simulink model "model"  (R2025b)
settings: Solver=FixedStepAuto  StartTime=0.0  StopTime=inf  FixedStep=0.01  RelTol=1e-3  EnableMultiTasking=on
libraries: GenericTarget x18, simulink x3
settings Model: Creator=Scythe  LastModifiedBy=damerius
settings SolverCC: ConcurrentTasks=on
settings DataIOCC: SaveOutput=off  SignalLogging=off  DSMLogging=off  SaveTime=off  ReturnWorkspaceOutputs=off
settings OptimizationCC: DefaultParameterBehavior=Inlined  EnhancedBackFolding=on  PassReuseOutputArgsAs=Individual arguments  ZeroExternalMemoryAtStartup=off  ZeroInternalMemoryAtStartup=off  SimCompilerOptimization=on  OptimizeBlockOrder=speed  DifferentSizesBufferReuse=on  OptimizationCustomize=off  EfficientTunableParamExpr=on
settings DebuggingCC: ParameterTunabilityLossMsg=error  UnconnectedInputMsg=warning  UnconnectedOutputMsg=warning  UnconnectedLineMsg=warning
settings HardwareCC: ProdBitPerLong=64.0  ProdHWDeviceType=Intel->x86-64 (Linux 64)  TargetBitPerLong=64.0  TargetBitPerPointer=64.0  TargetBitPerSizeT=64.0  TargetBitPerPtrDiffT=64.0  TargetLargestAtomicFloat=Float  TargetIntDivRoundTo=Zero  TargetEndianess=LittleEndian  TargetWordSize=64.0  TargetHWDeviceType=Intel->x86-64 (Linux 64)  ProdEqTarget=off
settings ModelReferenceCC: EnableRefExpFcnMdlSchedulingChecks=on
settings SFSimCC: SimGenImportedTypeDefs=on  SimTargetLang=C++  SimDLTargetLibrary=mkl-dnn
settings RTWCC: SystemTargetFile=ert.tlc  GenCodeOnly=on  PackageGeneratedCodeAndArtifacts=on  PackageName=PackNGo  TemplateMakefile=ert_default_tmf  Toolchain=CMake  DataTypeReplacement=CDataTypesFixedWidth  TargetLang=C++  Description=Embedded Coder
settings CodeAppCC: ForceParamTrailComments=on  IgnoreCustomStorageClasses=off  MaxIdLength=128.0  OperatorAnnotations=on  SimulinkDataObjDesc=on  SFDataObjDesc=on  InsertBlockDesc=on  StateflowObjectComments=on  MATLABSourceComments=on  UseSimReservedNames=on
settings ERTTargetCC: TargetOS=NativeThreadsExample  RootIOFormat=Structure reference  ERTCustomFileTemplate=example_file_process.tlc  IndentSize=4  NewlineStyle=LF  MaxLineWidth=256.0  MaxIdInt64=INT64_MAX  MinIdInt64=INT64_MIN  MaxIdUint64=UINT64_MAX  MaxIdInt32=INT32_MAX  MinIdInt32=INT32_MIN  MaxIdUint32=UINT32_MAX  MaxIdInt16=INT16_MAX  MinIdInt16=INT16_MIN  MaxIdUint16=UINT16_MAX  MaxIdInt8=INT8_MAX  MinIdInt8=INT8_MIN  MaxIdUint8=UINT8_MAX  DynamicArrayContainerType=coder::array  TargetLangStandard=C++20 (ISO)  CodeInterfacePackaging=C++ class  SubcomponentCodeInterfacePackaging=C++ class  SupportContinuousTime=on  SupportVariableSizeSignals=on

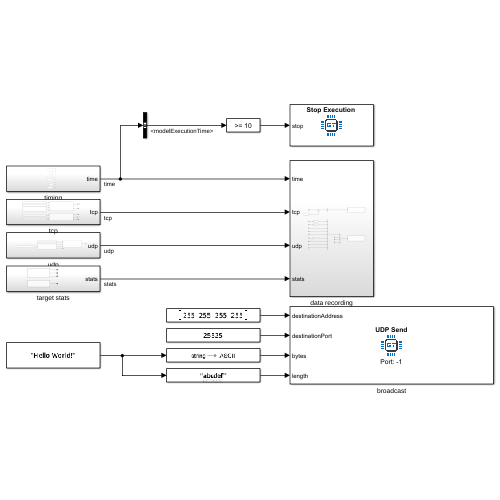
[thumbnail: Simulink's stored preview of the top-level diagram]
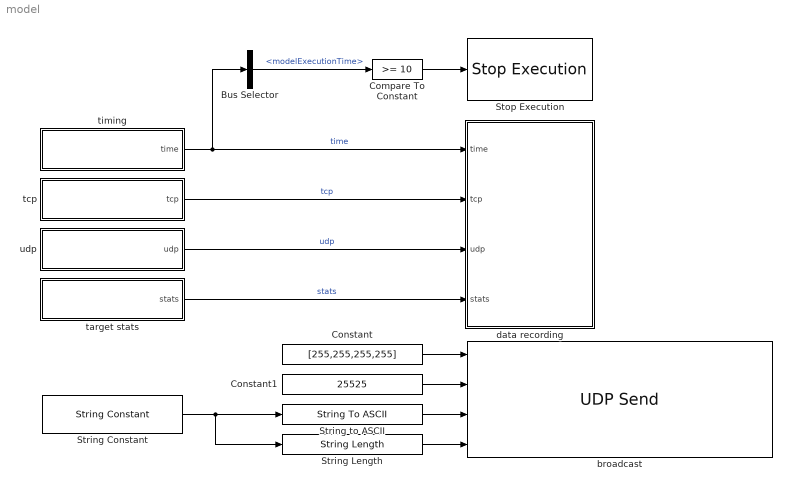
== system model ==
  Bus Selector : BusSelector  OutputSignals=modelExecutionTime
  Compare To Constant : simulink/Logic and Bit Operations/Compare To Constant  relop=>=  const=10  OutDataTypeStr=boolean
  Constant : Constant  Value=[255,255,255,255]  OutDataTypeStr=uint8
  Constant1 : Constant  Value=25525  OutDataTypeStr=uint16
  Stop Execution : GenericTarget/Interface/Stop Execution  SampleTime=0.01
      settings: SourceProductName=Generic Target
  String Constant : StringConstant  String="\"Hello World!\""
  String Length : StringLength  OutDataTypeStr=int32
  String to ASCII : StringToASCII  OutputVectorSize=63
  broadcast : GenericTarget/Interface/UDP Send  showDetails=off  localPort=-1  deviceName=''  multicastTTL=1  multicastInterfaceAddress=[0,0,0,0]  multicastAll=on  multicastLoop=on  socketPriority=6  allowBroadcast=on  allowZeroLengthMessage=off  SampleTime=1
      settings: SourceProductName=Generic Target
  data recording : Subsystem
  target stats : Subsystem
  tcp : Subsystem
  timing : Subsystem
  udp : Subsystem
  wires:
  target stats/1(stats) -> data recording/4(stats)  "stats"
  udp/1(udp) -> data recording/3(udp)  "udp"
  Bus Selector/1 -> Compare To Constant/1  "<modelExecutionTime>"
  timing/1(time) -> Bus Selector/1, data recording/1(time)  "time"
  Compare To Constant/1 -> Stop Execution/1
  Constant/1 -> broadcast/1
  Constant1/1 -> broadcast/2
  String to ASCII/1 -> broadcast/3
  String Length/1 -> broadcast/4
  String Constant/1 -> String Length/1, String to ASCII/1
  tcp/1(tcp) -> data recording/2(tcp)  "tcp"

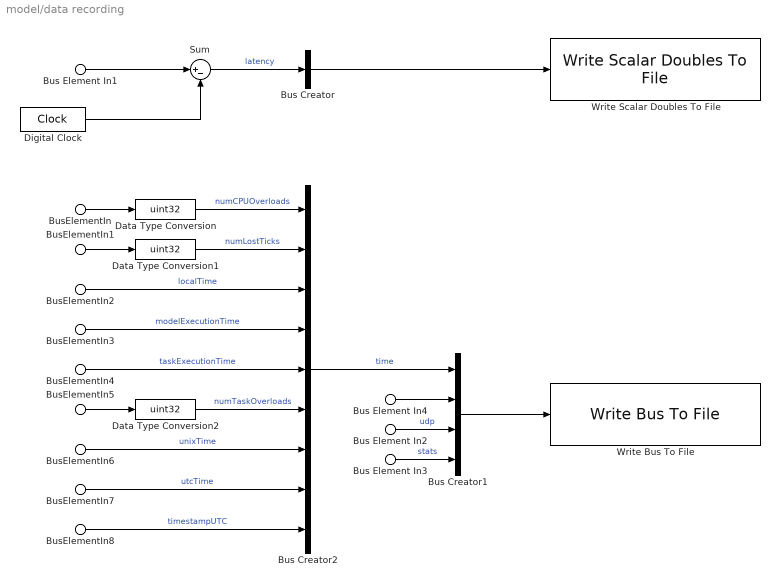
== system model/data recording ==
  Bus Element In1 : Inport  PortName=time  Element=modelExecutionTime
  BusElementIn3 : Inport  PortName=time  Element=modelExecutionTime
  BusElementIn : Inport  PortName=time  Element=numCPUOverloads
  BusElementIn1 : Inport  PortName=time  Element=numLostTicks
  BusElementIn2 : Inport  PortName=time  Element=localTime
  BusElementIn4 : Inport  PortName=time  Element=taskExecutionTime
  BusElementIn5 : Inport  PortName=time  Element=numTaskOverloads
  BusElementIn6 : Inport  PortName=time  Element=unixTime
  BusElementIn7 : Inport  PortName=time  Element=utcTime
  BusElementIn8 : Inport  PortName=time  Element=timestampUTC
  Bus Element In4 : Inport  Port=2  PortName=tcp
  Bus Element In2 : Inport  Port=3  PortName=udp
  Bus Element In3 : Inport  Port=4  PortName=stats
  Bus Creator : BusCreator  Inputs=1
  Bus Creator1 : BusCreator  Inputs=4
  Bus Creator2 : BusCreator  Inputs=9
  Data Type Conversion : DataTypeConversion  OutDataTypeStr=uint32  SaturateOnIntegerOverflow=off  RndMeth=Floor
  Data Type Conversion1 : DataTypeConversion  OutDataTypeStr=uint32  SaturateOnIntegerOverflow=off  RndMeth=Floor
  Data Type Conversion2 : DataTypeConversion  OutDataTypeStr=uint32  SaturateOnIntegerOverflow=off  RndMeth=Floor
  Digital Clock : DigitalClock  SampleTime=0.01
  Sum : Sum  Inputs=|+-
  Write Bus To File : GenericTarget/Interface/Write Bus To File  strID='bus'  numSamplesPerFile=0  threadPriority=30  writeFilesDuringSimulation=off  SampleTime=0.01  numBytesPerSample=305  strSignalNames='time.numCPUOverloads,time.numLostTicks,time.localTime.nanoseconds,time.localTime.second,time.localTime.minute,time.localTime.hour,time.localTime.mday,time.localTime.month,time.localTime.year,time.localTime.wday,time.localTime.yday,time.localTime.isdst,time.modelExecutionTime,time.taskExecutionTime,time.numTaskOverloads,time.unixTime,time.utcTime.nanoseconds,time.utcTime.second,time.utcTime.minute,time.utcTime.hour,time.utcTime.mday,time.utcTime.month,time.utcTime.year,time.utcTime.wday,time.utcTime.yday,time.utcTime.isdst,time.timestampUTC,tcp.tx_details.result,tcp.tx_details.lastErrorCode,tcp.tx_details.isConnected,tcp.rx_byte,tcp.rx_details.result,tcp.rx_details.lastErrorCode,tcp.rx_details.isConnected,udp.rx_details.sourceAddress,udp.rx_details.sourcePort,udp.rx_details.result,udp.rx_details.lastErrorCode,udp.tx_details.result,udp.tx_details.lastErrorCode,stats.applicationArguments.args,stats.applicationArguments.numCharacters,stats.applicationArguments.numArguments,stats.thermalZones'  strlenSignalNames=1002  strDimensions='[1],[1],[1],[1],[1],[1],[1],[1],[1],[1],[1],[1],[1],[1],[1],[1],[1],[1],[1],[1],[1],[1],[1],[1],[1],[1],[1],[1],[1],[1],[1],[1],[1],[1],[4],[1],[1],[1],[1],[1],[32 2],[2],[1],[8]'  strlenDimensions=178  strDataTypes='uint32,uint32,int32,int32,int32,int32,int32,int32,int32,int32,int32,int32,double,double,uint32,double,int32,int32,int32,int32,int32,int32,int32,int32,int32,int32,double,int32,int32,boolean,uint8,int32,int32,boolean,uint8,uint16,int32,int32,int32,int32,uint8,uint32,uint32,double'  strlenDataTypes=278
      settings: SourceProductName=Generic Target
  Write Scalar Doubles To File : GenericTarget/Interface/Write Scalar Doubles To File  strID='scalar_doubles'  numSamplesPerFile=0  threadPriority=30  writeFilesDuringSimulation=off  numSignals=1  signalNames=latency  numCharacters=7  SampleTime=0.01
      settings: SourceProductName=Generic Target
  wires:
  Bus Element In3/1 -> Bus Creator1/4  "stats"
  Bus Element In2/1 -> Bus Creator1/3  "udp"
  Bus Creator2/1 -> Bus Creator1/1  "time"
  BusElementIn8/1 -> Bus Creator2/9  "timestampUTC"
  BusElementIn7/1 -> Bus Creator2/8  "utcTime"
  BusElementIn6/1 -> Bus Creator2/7  "unixTime"
  Data Type Conversion2/1 -> Bus Creator2/6  "numTaskOverloads"
  BusElementIn4/1 -> Bus Creator2/5  "taskExecutionTime"
  BusElementIn3/1 -> Bus Creator2/4  "modelExecutionTime"
  BusElementIn2/1 -> Bus Creator2/3  "localTime"
  Data Type Conversion1/1 -> Bus Creator2/2  "numLostTicks"
  Data Type Conversion/1 -> Bus Creator2/1  "numCPUOverloads"
  BusElementIn5/1 -> Data Type Conversion2/1
  BusElementIn1/1 -> Data Type Conversion1/1
  BusElementIn/1 -> Data Type Conversion/1
  Bus Creator1/1 -> Write Bus To File/1
  Bus Creator/1 -> Write Scalar Doubles To File/1
  Sum/1 -> Bus Creator/1  "latency"
  Digital Clock/1 -> Sum/2
  Bus Element In1/1 -> Sum/1
  Bus Element In4/1 -> Bus Creator1/2

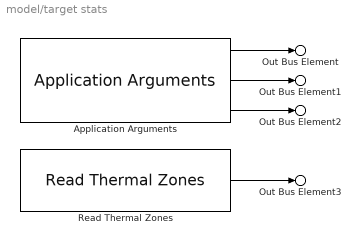
== system model/target stats ==
  Application Arguments : GenericTarget/Target Stats/Application Arguments  maxNumCharsPerArgument=32  maxNumArguments=2  SampleTime=0.01
      settings: SourceProductName=Generic Target
  Read Thermal Zones : GenericTarget/Target Stats/Read Thermal Zones  maxNumThermalZones=8  SampleTime=0.01
      settings: SourceProductName=Generic Target
  Out Bus Element : Outport  PortName=stats  Element=applicationArguments.args
  Out Bus Element1 : Outport  PortName=stats  Element=applicationArguments.numCharacters
  Out Bus Element2 : Outport  PortName=stats  Element=applicationArguments.numArguments
  Out Bus Element3 : Outport  PortName=stats  Element=thermalZones
  wires:
  Read Thermal Zones/1 -> Out Bus Element3/1
  Application Arguments/3 -> Out Bus Element2/1
  Application Arguments/2 -> Out Bus Element1/1
  Application Arguments/1 -> Out Bus Element/1

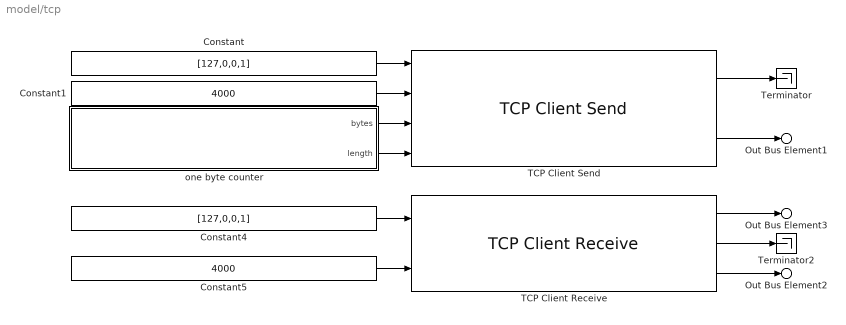
== system model/tcp ==
  Constant : Constant  Value=[127,0,0,1]  OutDataTypeStr=uint8
  Constant1 : Constant  Value=4000  OutDataTypeStr=uint16
  Constant4 : Constant  Value=[127,0,0,1]  OutDataTypeStr=uint8
  Constant5 : Constant  Value=4000  OutDataTypeStr=uint16
  TCP Client Receive : GenericTarget/Interface/TCP Client Receive  showDetails=on  manageConnection=off  localPort=0  deviceName=''  rxBufferSize=1  socketPriority=6  SampleTime=0.01
  TCP Client Send : GenericTarget/Interface/TCP Client Send  showDetails=on  manageConnection=on  localPort=0  deviceName=''  socketPriority=6  SampleTime=0.01
  Terminator : Terminator
  Terminator2 : Terminator
  one byte counter : Subsystem
  Out Bus Element1 : Outport  PortName=tcp  Element=tx_details
  Out Bus Element3 : Outport  PortName=tcp  Element=rx_byte
  Out Bus Element2 : Outport  PortName=tcp  Element=rx_details
  wires:
  TCP Client Send/2 -> Out Bus Element1/1
  Constant/1 -> TCP Client Send/1
  Constant1/1 -> TCP Client Send/2
  TCP Client Send/1 -> Terminator/1
  TCP Client Receive/1 -> Out Bus Element3/1
  TCP Client Receive/2 -> Terminator2/1
  Constant5/1 -> TCP Client Receive/2
  Constant4/1 -> TCP Client Receive/1
  TCP Client Receive/3 -> Out Bus Element2/1
  one byte counter/1(bytes) -> TCP Client Send/3
  one byte counter/2(length) -> TCP Client Send/4

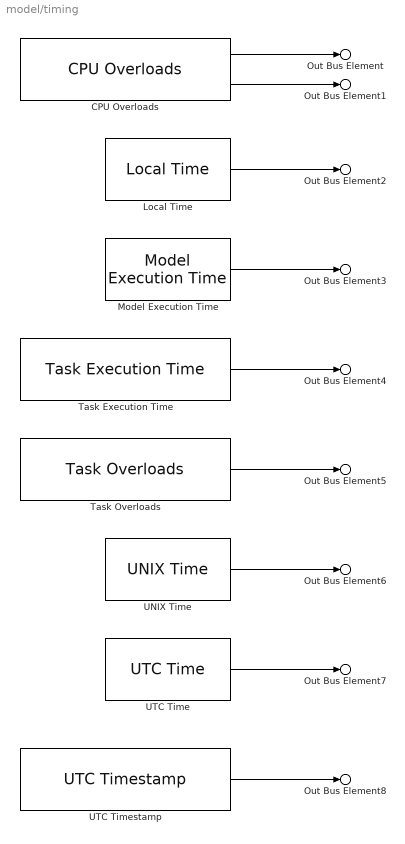
== system model/timing ==
  CPU Overloads : GenericTarget/Time/CPU Overloads  SampleTime=0.01
      settings: SourceProductName=Generic Target
  Local Time : GenericTarget/Time/Local Time  SampleTime=0.01
      settings: SourceProductName=Generic Target
  Model Execution Time : GenericTarget/Time/Model Execution Time  SampleTime=0.01
      settings: SourceProductName=Generic Target
  Task Execution Time : GenericTarget/Time/Task Execution Time  strTaskName='D1'  SampleTime=0.01
      settings: SourceProductName=Generic Target
  Task Overloads : GenericTarget/Time/Task Overloads  strTaskName='D1'  SampleTime=0.01
      settings: SourceProductName=Generic Target
  UNIX Time : GenericTarget/Time/UNIX Time  SampleTime=0.01
      settings: SourceProductName=Generic Target
  UTC Time : GenericTarget/Time/UTC Time  SampleTime=0.01
      settings: SourceProductName=Generic Target
  UTC Timestamp : GenericTarget/Time/UTC Timestamp  SampleTime=0.01
      settings: SourceProductName=Generic Target
  Out Bus Element : Outport  PortName=time  Element=numCPUOverloads
  Out Bus Element1 : Outport  PortName=time  Element=numLostTicks
  Out Bus Element2 : Outport  PortName=time  Element=localTime
  Out Bus Element3 : Outport  PortName=time  Element=modelExecutionTime
  Out Bus Element4 : Outport  PortName=time  Element=taskExecutionTime
  Out Bus Element5 : Outport  PortName=time  Element=numTaskOverloads
  Out Bus Element6 : Outport  PortName=time  Element=unixTime
  Out Bus Element7 : Outport  PortName=time  Element=utcTime
  Out Bus Element8 : Outport  PortName=time  Element=timestampUTC
  wires:
  UTC Timestamp/1 -> Out Bus Element8/1
  UTC Time/1 -> Out Bus Element7/1
  UNIX Time/1 -> Out Bus Element6/1
  Task Overloads/1 -> Out Bus Element5/1
  Task Execution Time/1 -> Out Bus Element4/1
  Model Execution Time/1 -> Out Bus Element3/1
  Local Time/1 -> Out Bus Element2/1
  CPU Overloads/2 -> Out Bus Element1/1
  CPU Overloads/1 -> Out Bus Element/1

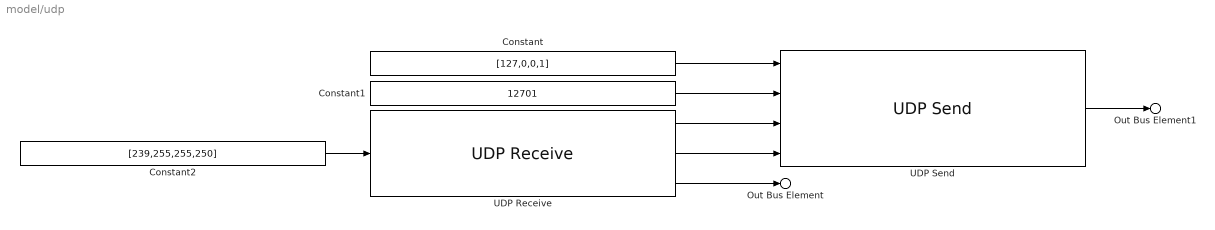
== system model/udp ==
  Constant : Constant  Value=[127,0,0,1]  OutDataTypeStr=uint8
  Constant1 : Constant  Value=12701  OutDataTypeStr=uint16
  Constant2 : Constant  Value=[239,255,255,250]  OutDataTypeStr=uint8
  UDP Receive : GenericTarget/Interface/UDP Receive  showDetails=on  localPort=1900  deviceName=''  rxBufferSize=2048  multicastGroupSource=external  multicastGroup=[0,0,0,0]  multicastTTL=1  multicastInterfaceAddress=[0,0,0,0]  multicastAll=on  multicastLoop=on  socketPriority=6  allowBroadcast=off  allowZeroLengthMessage=off  fetchAll=on  SampleTime=0.01
      settings: SourceProductName=Generic Target
  UDP Send : GenericTarget/Interface/UDP Send  showDetails=on  localPort=0  deviceName=''  multicastTTL=1  multicastInterfaceAddress=[0,0,0,0]  multicastAll=on  multicastLoop=on  socketPriority=6  allowBroadcast=off  allowZeroLengthMessage=off  SampleTime=0.01
      settings: SourceProductName=Generic Target
  Out Bus Element : Outport  PortName=udp  Element=rx_details
  Out Bus Element1 : Outport  PortName=udp  Element=tx_details
  wires:
  Constant2/1 -> UDP Receive/1
  UDP Send/1 -> Out Bus Element1/1
  UDP Receive/3 -> Out Bus Element/1
  Constant1/1 -> UDP Send/2
  Constant/1 -> UDP Send/1
  UDP Receive/2 -> UDP Send/4
  UDP Receive/1 -> UDP Send/3

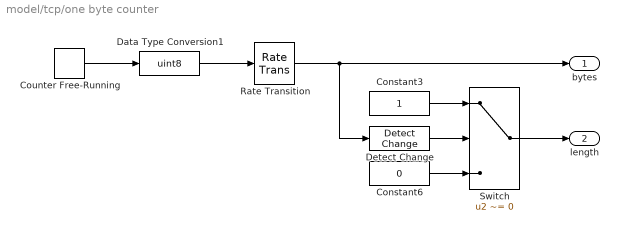
== system model/tcp/one byte counter ==
  Constant3 : Constant  OutDataTypeStr=int32
  Constant6 : Constant  Value=0  OutDataTypeStr=int32
  Counter Free-Running : simulink/Sources/Counter Free-Running  NumBits=8  tsamp=1
  Data Type Conversion1 : DataTypeConversion  OutDataTypeStr=uint8  SaturateOnIntegerOverflow=off  RndMeth=Floor
  Detect Change : simulink/Logic and Bit Operations/Detect Change  vinit=0  OutDataTypeStr=boolean
  Rate Transition : RateTransition  Deterministic=off  OutPortSampleTime=0.01
  Switch : Switch  Criteria=u2 ~= 0  SaturateOnIntegerOverflow=off  InputSameDT=off
  bytes : Outport
  length : Outport  Port=2
  wires:
  Detect Change/1 -> Switch/2
  Rate Transition/1 -> bytes/1, Detect Change/1
  Counter Free-Running/1 -> Data Type Conversion1/1
  Constant6/1 -> Switch/3
  Constant3/1 -> Switch/1
  Data Type Conversion1/1 -> Rate Transition/1
  Switch/1 -> length/1
